simulink model "test3"  (R2016a)
settings: Solver=FixedStepDiscrete  StartTime=0.0  StopTime=30.0  FixedStep=5e-6  RelTol=1e-3
libraries: powerlib x20, powerlib_meascontrol x1, simulink x1
settings Model: Creator=Dang Khoa  LastModifiedBy=Dang Khoa

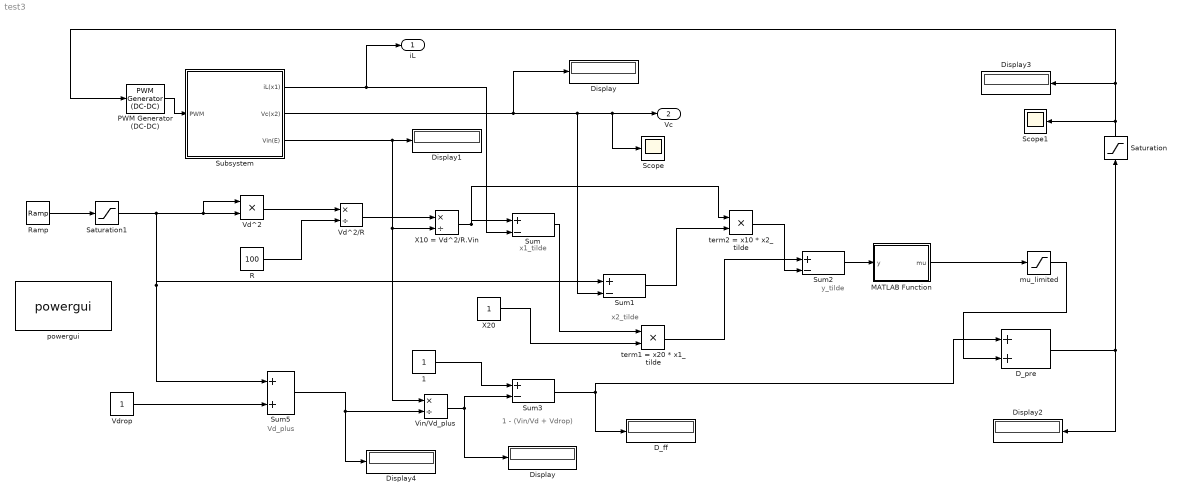
== system test3 ==
  note: Vd_plus
  note: 1 - (Vin/Vd + Vdrop)
  note: x1_tilde
  note: x2_tilde
  note: y_tilde
  "1 " : Constant
  D_ff : Display
  D_pre : Sum
  Display{,1..4} (5 alike) : Display
  "Display " : Display
  MATLAB Function : MATLAB Function  TreatAsAtomicUnit=on
  PWM Generator (DC-DC) : powerlib_meascontrol/Pulse & Signal Generators/PWM Generator (DC-DC)  Fsw=1/20000  Ts=5e-06
  R : Constant  Value=100
  Ramp : simulink/Sources/Ramp  slope=200  start=0  X0=0
  Saturation : Saturate  UpperLimit=1  LowerLimit=0
  Saturation1 : Saturate  UpperLimit=20  LowerLimit=0
  Scope : Scope
  Scope1 : Scope
  Subsystem : Subsystem
  Sum : Sum  Inputs=|+-
  Sum1 : Sum  Inputs=|+-
  Sum2 : Sum  Inputs=|+-
  Sum3 : Sum  Inputs=+-
  Sum5 : Sum
  Vd^2 : Product
  Vd^2/R : Product  Inputs=*/
  Vdrop : Constant  SampleTime=5e-6
  Vin/Vd_plus : Product  Inputs=*/
  X10 = Vd^2/R.Vin : Product  Inputs=*/
  X20 : Constant
  mu_limited : Saturate  UpperLimit=0.3  LowerLimit=-0.3
  powergui : powerlib/powergui  Priority=1  SimulationMode=Discrete  SolverType=Tustin/Backward Euler (TBE)  SampleTime=5e-6  frequency=60  SPID=off  DisableSnubberDevices=off  DisableRonSwitches=off  DisableVfSwitches=off  SwTol=0  DisplayEquations=off  Interpol=off  ExternalGateDelay=off  methode=off  Ts=10  FunctionMessages=off  echomessages=off  HookPort=off  EnableUseOfTLC=off  x0status=blocks  frequencyindice=0  Pbase=100e6  ErrMax=1e-4  Iterations=50  UnitsV=kV  UnitsW=MW  buscounter=0  RestoreLinks=warning  ResistiveCurrentMeasurement=off  Frange=[0:2:500]  Ylog=off  Xlog=on  ShowGrid=off  save=off  variable=ZData  structure=0  ZoomFFT=off  StartTime=0.0  cycles=1  DisplayStyle=1  fundamental=60  FreqAxis=off  MaxFrequency=1000  frequencyindicesteady=1  RmsSteady=1  display=off
  term1 = x20 * x1_tilde : Product
  term2 = x10 * x2_tilde : Product
  iL : Outport
  Vc : Outport  Port=2
  wires:
  PWM Generator (DC-DC)/1 -> Subsystem/1(PWM)
  Ramp/1 -> Saturation1/1
  Vd^2/1 -> Vd^2/R/1
  R/1 -> Vd^2/R/2
  Vd^2/R/1 -> X10 = Vd^2/R.Vin/1
  Subsystem/3(Vin(E)) -> Display1/1, Vin/Vd_plus/1, X10 = Vd^2/R.Vin/2
  X10 = Vd^2/R.Vin/1 -> term2 = x10 * x2_tilde/1, Sum/1
  Subsystem/2(Vc(x2)) -> Display/1, Scope/1, Vc/1, Sum1/2
  Sum/1 -> term1 = x20 * x1_tilde/1
  term1 = x20 * x1_tilde/1 -> Sum2/1
  term2 = x10 * x2_tilde/1 -> Sum2/2
  "1 "/1 -> Sum3/1
  Vin/Vd_plus/1 -> "Display "/1, Sum3/2
  Sum3/1 -> D_pre/1, D_ff/1
  Sum2/1 -> MATLAB Function/1(y)
  Vdrop/1 -> Sum5/2
  Sum5/1 -> Display4/1, Vin/Vd_plus/2
  D_pre/1 -> Display2/1, Saturation/1
  Saturation/1 -> Display3/1, PWM Generator (DC-DC)/1, Scope1/1
  Subsystem/1(iL(x1)) -> iL/1, Sum/2
  MATLAB Function/1(mu) -> mu_limited/1
  Saturation1/1 -> Sum1/1, Sum5/1, Vd^2/1, Vd^2/2
  mu_limited/1 -> D_pre/2
  X20/1 -> term1 = x20 * x1_tilde/2
  Sum1/1 -> term2 = x10 * x2_tilde/2

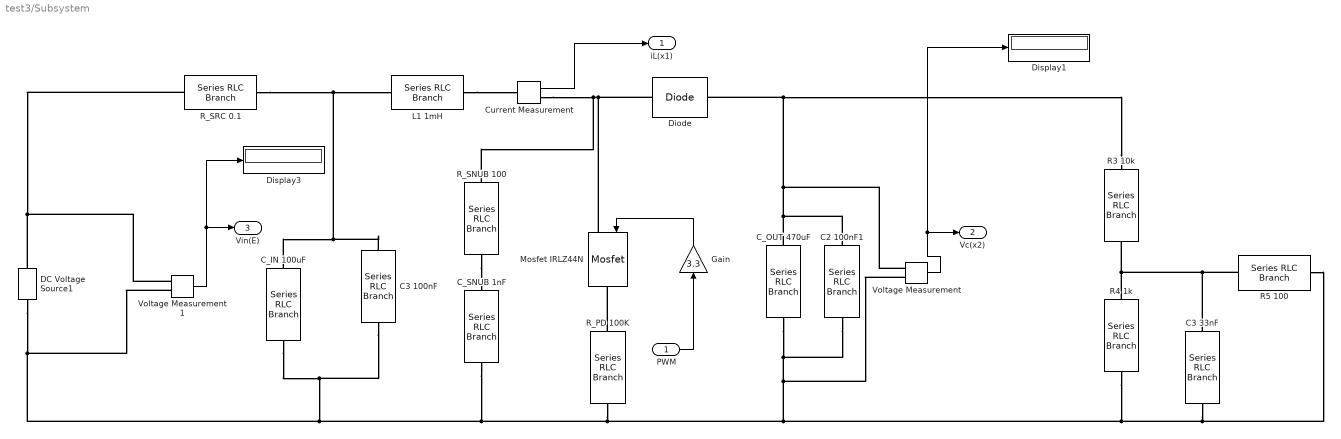
== system test3/Subsystem ==
  PWM : Inport
  C2 100nF1 : powerlib/Elements/Series RLC Branch  LConnTagsString=__new0  RConnTagsString=__new0  BranchType=C  Resistance=1  Inductance=1e-3  SetiL0=off  InitialCurrent=0  Capacitance=100e-9  Setx0=off  InitialVoltage=0  Measurements=None
  C3 100nF : powerlib/Elements/Series RLC Branch  LConnTagsString=__new0  RConnTagsString=__new0  BranchType=C  Resistance=1  Inductance=1e-3  SetiL0=off  InitialCurrent=0  Capacitance=100e-9  Setx0=off  InitialVoltage=0  Measurements=None
  C3 33nF : powerlib/Elements/Series RLC Branch  LConnTagsString=__new0  RConnTagsString=__new0  BranchType=C  Resistance=1  Inductance=1e-3  SetiL0=off  InitialCurrent=0  Capacitance=33e-9  Setx0=off  InitialVoltage=0  Measurements=None
  C_IN 100uF : powerlib/Elements/Series RLC Branch  LConnTagsString=__new0  RConnTagsString=__new0  BranchType=C  Resistance=1  Inductance=1e-3  SetiL0=off  InitialCurrent=0  Capacitance=100e-6  Setx0=off  InitialVoltage=0  Measurements=None
  C_OUT 470uF : powerlib/Elements/Series RLC Branch  LConnTagsString=__new0  RConnTagsString=__new0  BranchType=C  Resistance=1  Inductance=1e-3  SetiL0=off  InitialCurrent=0  Capacitance=470e-6  Setx0=off  InitialVoltage=0  Measurements=None
  C_SNUB 1nF : powerlib/Elements/Series RLC Branch  LConnTagsString=__new0  RConnTagsString=__new0  BranchType=C  Resistance=1  Inductance=1e-3  SetiL0=off  InitialCurrent=0  Capacitance=1e-9  Setx0=off  InitialVoltage=0  Measurements=None
  Current Measurement : powerlib/Measurements/Current Measurement  PhasorSimulation=off  OutputType=Complex  PSBequivalent=0
  DC Voltage Source1 : powerlib/Electrical Sources/DC Voltage Source  Amplitude=15  Measurements=None
  "Diode " : powerlib/Power Electronics/Diode  Ron=0.05  Lon=0  Vf=1  IC=0  UseSnubber=off  Rs=500  Cs=250e-9  Measurements=off
  Display1 : Display
  Display3 : Display
  Gain : Gain  Gain=3.3
  L1 1mH : powerlib/Elements/Series RLC Branch  LConnTagsString=__new0  RConnTagsString=__new0  BranchType=L  Resistance=1  Inductance=0.001  SetiL0=off  InitialCurrent=0  Capacitance=1e-6  Setx0=off  InitialVoltage=0  Measurements=None
  Mosfet IRLZ44N : powerlib/Power Electronics/Mosfet  Ron=0.03  Lon=0  Rd=0.05  Vfd=0.09  IC=0  Rs=inf  Cs=inf  Measurements=off
  R3 10k : powerlib/Elements/Series RLC Branch  LConnTagsString=__new0  RConnTagsString=__new0  BranchType=R  Resistance=100000  Inductance=1e-3  SetiL0=off  InitialCurrent=0  Capacitance=1e-6  Setx0=off  InitialVoltage=0  Measurements=None
  R4 1k : powerlib/Elements/Series RLC Branch  LConnTagsString=__new0  RConnTagsString=__new0  BranchType=R  Resistance=10000  Inductance=1e-3  SetiL0=off  InitialCurrent=0  Capacitance=1e-6  Setx0=off  InitialVoltage=0  Measurements=None
  R5 100 : powerlib/Elements/Series RLC Branch  LConnTagsString=__new0  RConnTagsString=__new0  BranchType=R  Resistance=100  Inductance=1e-3  SetiL0=off  InitialCurrent=0  Capacitance=1e-6  Setx0=off  InitialVoltage=0  Measurements=None
  R_PD 100K : powerlib/Elements/Series RLC Branch  LConnTagsString=__new0  RConnTagsString=__new0  BranchType=R  Resistance=100000  Inductance=1e-3  SetiL0=off  InitialCurrent=0  Capacitance=1e-6  Setx0=off  InitialVoltage=0  Measurements=None
  R_SNUB 100 : powerlib/Elements/Series RLC Branch  LConnTagsString=__new0  RConnTagsString=__new0  BranchType=R  Resistance=100  Inductance=1e-3  SetiL0=off  InitialCurrent=0  Capacitance=1e-6  Setx0=off  InitialVoltage=0  Measurements=None
  R_SRC 0.1 : powerlib/Elements/Series RLC Branch  LConnTagsString=__new0  RConnTagsString=__new0  BranchType=R  Resistance=0.1  Inductance=1e-3  SetiL0=off  InitialCurrent=0  Capacitance=1e-6  Setx0=off  InitialVoltage=0  Measurements=None
  Voltage Measurement : powerlib/Measurements/Voltage Measurement  PhasorSimulation=off  OutputType=Complex  PSBequivalent=0
  Voltage Measurement1 : powerlib/Measurements/Voltage Measurement  PhasorSimulation=off  OutputType=Complex  PSBequivalent=0
  iL(x1) : Outport
  Vc(x2) : Outport  Port=2
  Vin(E) : Outport  Port=3
  wires:
  Voltage Measurement/1 -> Display1/1, Vc(x2)/1
  Current Measurement/1 -> iL(x1)/1
  Voltage Measurement1/1 -> Display3/1, Vin(E)/1
  PWM/1 -> Gain/1
  Gain/1 -> Mosfet IRLZ44N/1
  connections:
  R4 1k/LConn1 -- C3 33nF/LConn1 -- R5 100/LConn1 -- R3 10k/RConn1
  Voltage Measurement1/LConn2 -- DC Voltage Source1/LConn1 -- C_SNUB 1nF/RConn1 -- R4 1k/RConn1 -- C3 33nF/RConn1 -- R5 100/RConn1 -- Voltage Measurement/LConn2 -- C_OUT 470uF/RConn1 -- C2 100nF1/RConn1 -- R_PD 100K/RConn1 -- C3 100nF/RConn1 -- C_IN 100uF/RConn1
  Current Measurement/RConn1 -- "Diode "/LConn1 -- Mosfet IRLZ44N/LConn1 -- R_SNUB 100/LConn1
  R3 10k/LConn1 -- C2 100nF1/LConn1 -- C_OUT 470uF/LConn1 -- Voltage Measurement/LConn1 -- "Diode "/RConn1
  C_IN 100uF/LConn1 -- C3 100nF/LConn1 -- R_SRC 0.1/RConn1 -- L1 1mH/LConn1
  L1 1mH/RConn1 -- Current Measurement/LConn1
  Voltage Measurement1/LConn1 -- R_SRC 0.1/LConn1 -- DC Voltage Source1/RConn1
  R_PD 100K/LConn1 -- Mosfet IRLZ44N/RConn1
  R_SNUB 100/RConn1 -- C_SNUB 1nF/LConn1

== matlab function test3/MATLAB Function ==
  data: y input; mu output
function mu = PBCphi(y)
% y = x20*x1_tilde - x10*x2_tilde, x20 = 1
% trong block PBCphi
a1 = 0.06;
a2 = 0.012;
a3 = 0.003;
mu = -(a1*y + a2*y.^3 + a3*y.^5);   % DẤU ÂM đúng Cách A
end
